simulink model "FOSWEC"  (R2014b)
settings: Solver=ode45  StartTime=0.0  StopTime=10.0  RelTol=1e-3
undefined symbols (not defined in the file or in its folder): body, constraint, pto
libraries: WECSim_Lib x7
settings Model: Creator=cmichel  LastModifiedBy=cmichel

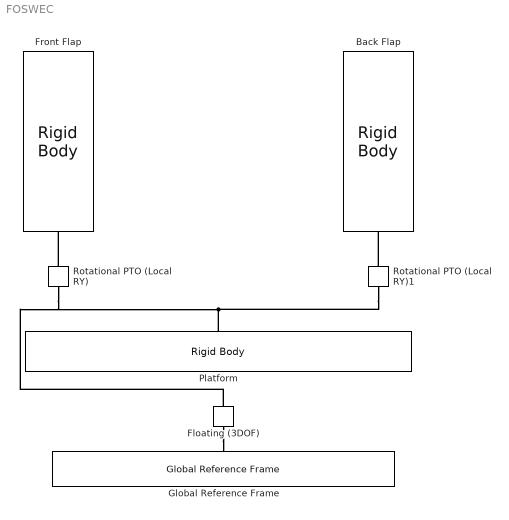
== system FOSWEC ==
  Back Flap : WECSim_Lib/Body Elements/Rigid Body  body=body(3)
      settings: AttributesFormatString=%<body>
  Floating (3DOF) : WECSim_Lib/Constraints/Floating (3DOF)  constraint=constraint(1)
      settings: AttributesFormatString=%<constraint>
  Front Flap : WECSim_Lib/Body Elements/Rigid Body  body=body(2)
      settings: AttributesFormatString=%<body>
  Global Reference Frame : WECSim_Lib/Frames/Global Reference Frame  waves=waves  simu=simu
  Platform : WECSim_Lib/Body Elements/Rigid Body  body=body(1)
      settings: AttributesFormatString=%<body>
  Rotational PTO (Local RY) : WECSim_Lib/PTOs/Rotational PTO (Local RY)  pto=pto(1)
      settings: AttributesFormatString=%<pto>
  Rotational PTO (Local RY)1 : WECSim_Lib/PTOs/Rotational PTO (Local RY)  pto=pto(2)
      settings: AttributesFormatString=%<pto>
  connections:
  Rotational PTO (Local RY)/RConn1 -- Front Flap/RConn1
  Rotational PTO (Local RY)1/RConn1 -- Back Flap/RConn1
  Platform/RConn1 -- Rotational PTO (Local RY)1/LConn1 -- Floating (3DOF)/RConn1 -- Rotational PTO (Local RY)/LConn1
  Floating (3DOF)/LConn1 -- Global Reference Frame/RConn1
